simulink model "open_loop_sp_NPC"  (R2013a)
settings: Solver=FixedStepDiscrete  SolverMode=SingleTasking  StartTime=0.0  StopTime=5  FixedStep=Ts  RelTol=1e-3
InitFcn:
  | Ts = 5e-5
  | R = 0.28
  | L = 0.1
libraries: powerlib x10, simulink x4, powerlib_meascontrol x4
settings Model: Creator=Daniel  LastModifiedBy=Daniel

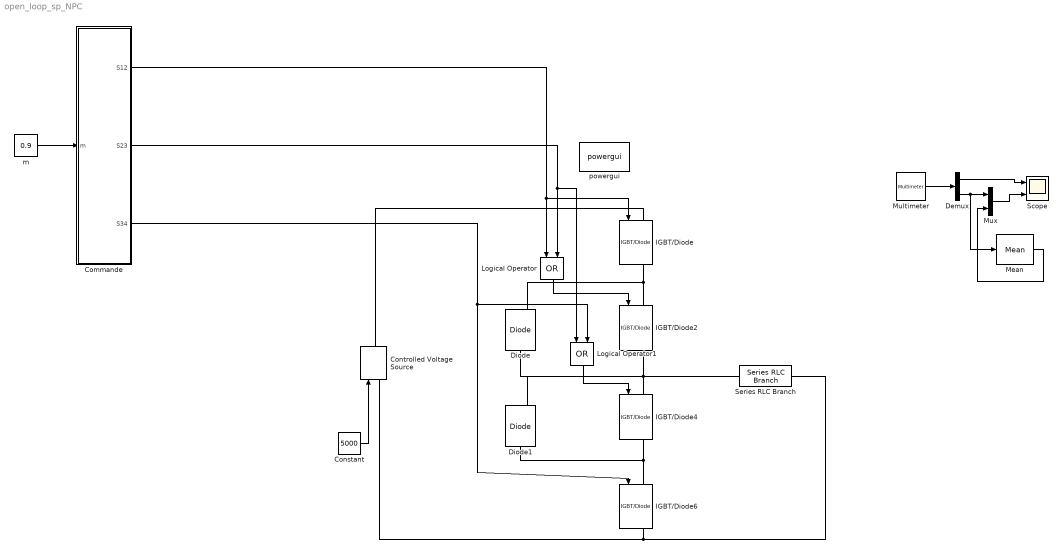
== system open_loop_sp_NPC ==
  Commande : Subsystem  SystemSampleTime=Ts
      settings: MinAlgLoopOccurrences=on
  Constant : Constant  Value=5000  SampleTime=Ts
  Controlled Voltage Source : powerlib/Electrical Sources/Controlled Voltage Source  Initialize=on  Source_Type=AC  Amplitude=0  Phase=0  Frequency=0  Measurements=None
  Demux : Demux  Outputs=2
  Diode : powerlib/Power Electronics/Diode  Ron=0.001  Lon=0  Vf=0.8  IC=0  UseSnubber=off  Rs=500  Cs=250e-9  Measurements=on
  Diode1 : powerlib/Power Electronics/Diode  Ron=0.001  Lon=0  Vf=0.8  IC=0  UseSnubber=off  Rs=500  Cs=250e-9  Measurements=on
  IGBT/Diode{,2,4,6} (4 alike) : powerlib/Power Electronics/IGBT//Diode  Ron=1e-3  Rs=1e5  Cs=inf  Measurements=on
  Logical Operator : Logic  Operator=OR  AllPortsSameDT=off  OutDataTypeStr=boolean
  Logical Operator1 : Logic  Operator=OR  AllPortsSameDT=off  OutDataTypeStr=boolean
  Mean : powerlib_meascontrol/Measurements/Mean  Freq=1000  Vinit=0  Ts=Ts
  Multimeter : powerlib/Measurements/Multimeter  PhasorSimulation=off  OutputType=Complex  sel=[2 1]  L=2  Gain=[1 1]  yselected={'Ib: Series RLC Branch','Ub: Series RLC Branch'};  PSBOutputType=1  PSBequivalent=0  AxesSetting=[0,0.1,-100,100]  Display=0  SavedBlockNames=-11
  Mux : Mux  Inputs=2
  Scope : Scope  NumInputPorts=2
      settings: YMin=-5~-5  YMax=5~5
  Series RLC Branch : powerlib/Elements/Series RLC Branch  LConnTagsString=__new0  RConnTagsString=__new0  BranchType=RL  Resistance=R  Inductance=L  SetiL0=off  InitialCurrent=0  Capacitance=1e-6  Setx0=off  InitialVoltage=0  Measurements=Branch voltage and current
  m : Constant  Value=0.9  SampleTime=Ts
  powergui : powerlib/powergui  Priority=1  SimulationMode=Discrete  SolverType=Tustin  SampleTime=50e-6  frequency=60  SPID=off  DisableSnubberDevices=off  DisableRonSwitches=off  DisableVfSwitches=off  SwTol=0  Interpol=off  DisplayEquations=off  frequencyindice=0  Pbase=100e6  ErrMax=1e-4  Iterations=50  UnitsV=kV  UnitsW=MW  FunctionMessages=off  echomessages=off  HookPort=off  EnableUseOfTLC=off  x0status=blocks  RestoreLinks=warning  ResistiveCurrentMeasurement=off  Frange=[0:2:500]  Ylog=off  Xlog=on  ShowGrid=off  save=off  variable=ZData  ZoomFFT=off  StartTime=0.0  cycles=1  DisplayStyle=1  fundamental=60  FreqAxis=off  MaxFrequency=1000  frequencyindicesteady=1  RmsSteady=1  display=off  Ts=0  methode=off
  wires:
  Constant/1 -> Controlled Voltage Source/1
  m/1 -> Commande/1(m)
  Commande/1(S12) -> IGBT/Diode/1, Logical Operator/1
  Commande/2(S23) -> Logical Operator1/1, Logical Operator/2
  Logical Operator/1 -> IGBT/Diode2/1
  Commande/3(S34) -> IGBT/Diode6/1, Logical Operator1/2
  Logical Operator1/1 -> IGBT/Diode4/1
  Multimeter/1 -> Demux/1
  Demux/2 -> Mean/1, Mux/1
  Mean/1 -> Mux/2
  Demux/1 -> Scope/1
  Mux/1 -> Scope/2
  connections:
  IGBT/Diode2/RConn1 -- Diode/LConn1 -- Diode1/RConn1 -- Series RLC Branch/LConn1 -- IGBT/Diode4/LConn1
  IGBT/Diode6/LConn1 -- Diode1/LConn1 -- IGBT/Diode4/RConn1
  IGBT/Diode6/RConn1 -- Series RLC Branch/RConn1 -- Controlled Voltage Source/LConn1
  IGBT/Diode2/LConn1 -- Diode/RConn1 -- IGBT/Diode/RConn1
  IGBT/Diode/LConn1 -- Controlled Voltage Source/RConn1

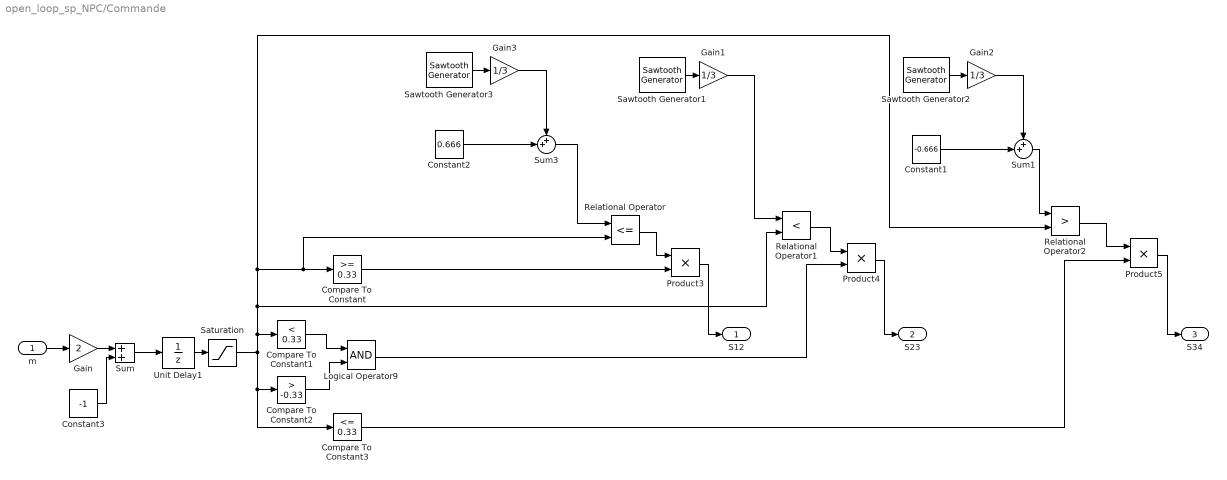
== system open_loop_sp_NPC/Commande ==
  m : Inport
  Compare To Constant : simulink/Logic and Bit Operations/Compare To Constant  relop=>=  const=0.33  OutDataTypeStr=boolean
  Compare To Constant1 : simulink/Logic and Bit Operations/Compare To Constant  relop=<  const=0.33  OutDataTypeStr=boolean
  Compare To Constant2 : simulink/Logic and Bit Operations/Compare To Constant  relop=>  const=-0.33  OutDataTypeStr=boolean
  Compare To Constant3 : simulink/Logic and Bit Operations/Compare To Constant  relop=<=  const=0.33  OutDataTypeStr=boolean
  Constant1 : Constant  Value=-0.666  SampleTime=Ts
  Constant2 : Constant  Value=0.666  SampleTime=Ts
  Constant3 : Constant  Value=-1  SampleTime=Ts
  Gain : Gain  Gain=2
  Gain1 : Gain  Gain=1/3  SampleTime=Ts
  Gain2 : Gain  Gain=1/3  SampleTime=Ts
  Gain3 : Gain  Gain=1/3  SampleTime=Ts
  Logical Operator9 : Logic  AllPortsSameDT=off  OutDataTypeStr=boolean  SampleTime=Ts
  Product3 : Product  SampleTime=Ts
  Product4 : Product  SampleTime=Ts
  Product5 : Product  SampleTime=Ts
  Relational Operator : RelationalOperator  Operator=<=  OutDataTypeStr=boolean  SampleTime=Ts
  Relational Operator1 : RelationalOperator  Operator=<  OutDataTypeStr=boolean  SampleTime=Ts
  Relational Operator2 : RelationalOperator  Operator=>  OutDataTypeStr=boolean  SampleTime=Ts
  Saturation : Saturate  UpperLimit=1  LowerLimit=-1
  Sawtooth Generator1 : powerlib_meascontrol/Pulse & Signal Generators/Sawtooth Generator  Freq=1e3  Phase=0  Ts=Ts
  Sawtooth Generator2 : powerlib_meascontrol/Pulse & Signal Generators/Sawtooth Generator  Freq=1e3  Phase=0  Ts=Ts
  Sawtooth Generator3 : powerlib_meascontrol/Pulse & Signal Generators/Sawtooth Generator  Freq=1e3  Phase=0  Ts=Ts
  Sum : Sum  SampleTime=Ts
  Sum1 : Sum  Inputs=++|
  Sum3 : Sum  Inputs=++|
  Unit Delay1 : UnitDelay  SampleTime=-1
  S12 : Outport
  S23 : Outport  Port=2
  S34 : Outport  Port=3
  wires:
  Constant1/1 -> Sum1/2
  Sawtooth Generator1/1 -> Gain1/1
  Gain2/1 -> Sum1/1
  Sawtooth Generator2/1 -> Gain2/1
  Compare To Constant/1 -> Product3/2
  Compare To Constant3/1 -> Product5/2
  Unit Delay1/1 -> Saturation/1
  Gain1/1 -> Relational Operator1/1
  Sum1/1 -> Relational Operator2/1
  Sum3/1 -> Relational Operator/1
  Relational Operator/1 -> Product3/1
  Relational Operator1/1 -> Product4/1
  Relational Operator2/1 -> Product5/1
  Constant2/1 -> Sum3/2
  Gain3/1 -> Sum3/1
  Sawtooth Generator3/1 -> Gain3/1
  Compare To Constant1/1 -> Logical Operator9/1
  Compare To Constant2/1 -> Logical Operator9/2
  Logical Operator9/1 -> Product4/2
  Product3/1 -> S12/1
  Product4/1 -> S23/1
  Product5/1 -> S34/1
  m/1 -> Gain/1
  Gain/1 -> Sum/1
  Constant3/1 -> Sum/2
  Sum/1 -> Unit Delay1/1
  Saturation/1 -> Relational Operator2/2, Relational Operator/2, Compare To Constant/1, Relational Operator1/2, Compare To Constant1/1, Compare To Constant2/1, Compare To Constant3/1
